simulink model "PathFollowing_4_29"  (R2023b)
settings: Solver=FixedStepAuto  StartTime=0  StopTime=inf  FixedStep=0.01  RelTol=1e-3
InitFcn:
  | InitParam_cs;
StopFcn:
  | plotTrack;
values from neighbouring files (symbols this model uses):
  B0 = [0,-30]    [InitParam_cs.m]
  lamda = 0.2573    [main.m]
  P0 = [0,0]    [InitParam_cs.m]    (also in SetWaypoints.m)
  u_c = 0.1    [main.m]
  U_d = i    [main.m]
  v_c = 0.1    [main.m]
  V_w = 1    [main.m]
  w_e1 = 0.8    [main.m]
  w_e2 = 0.8    [main.m]
  w_e6 = 0.8    [main.m]
  Waypoints = [100 0;200 0]    [InitParam_cs.m]    (also in SetWaypoints.m = [80 0;120 0])
  WPNum = size(Waypoints,1)    [InitParam_cs.m]    (also in SetWaypoints.m)
  Yaw0 = 0    [InitParam_cs.m]    (also in SetWaypoints.m)
libraries: simulink x9, cstblocks x3, slpidlib x2
settings Model: Creator=53549  LastModifiedBy=Xue
settings SolverCC: AlgebraicLoopSolver=TrustRegion
settings DataIOCC: SaveFormat=StructureWithTime  ReturnWorkspaceOutputs=off
settings OptimizationCC: BlockReduction=off  BufferReuse=off
settings DebuggingCC: AlgebraicLoopMsg=none  ArithmeticOperatorsInVariantConditions=warning
settings ModelReferenceCC: EnableRefExpFcnMdlSchedulingChecks=on
settings SFSimCC: SimUseLocalCustomCode=off  CustomCodeUndefinedFunction=UseInterfaceOnly
settings RTWCC: RTWUseLocalCustomCode=off  DLArmComputeVersion=19.05
settings CodeAppCC: StateflowObjectComments=on

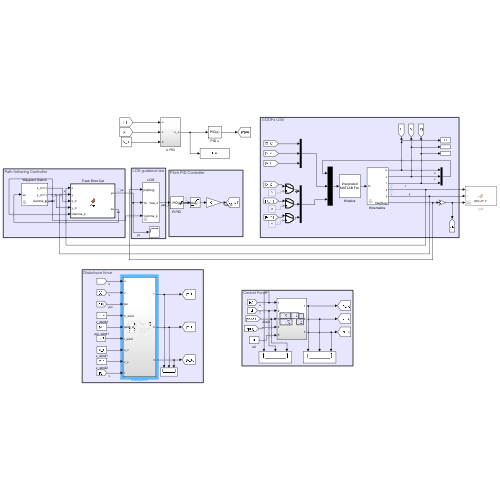
[thumbnail: Simulink's stored preview of the top-level diagram]
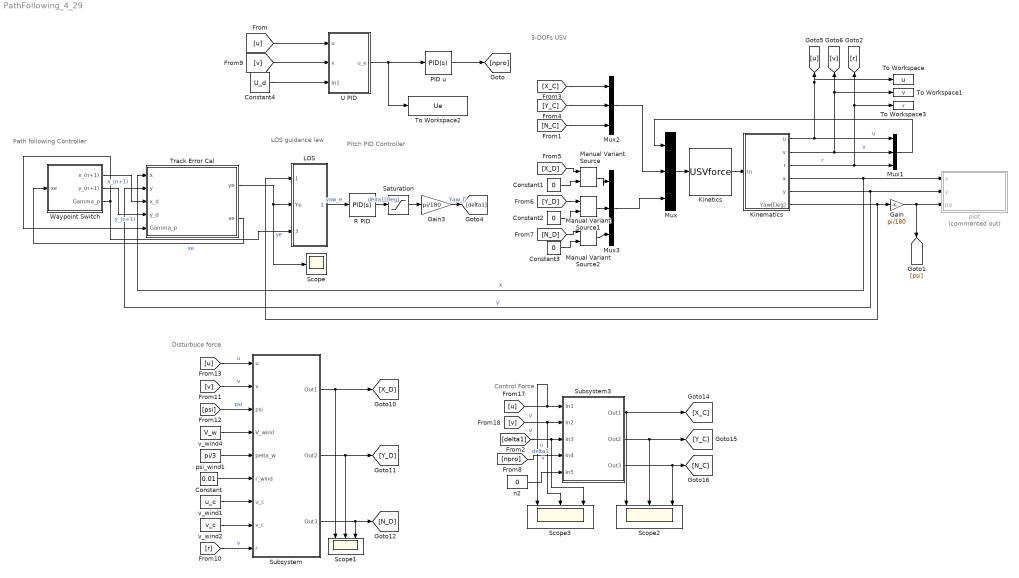
== system PathFollowing_4_29 ==
  note: LOS guidance law
  note: Disturbuce force
  note: v
  note: v
  note: Path following Controller
  note: 3-DOFs USV
  note: Control Force
  note: Pitch PID Controller
  Constant : Constant  Value=0.01
  Constant1 : Constant  Value=0
  Constant2 : Constant  Value=0
  Constant3 : Constant  Value=0
  Constant4 : Constant  Value=U_d
  Gain : Gain  Gain=pi/180
  Gain3 : Gain  Gain=pi/180
  "Kinematics " : Subsystem  mask{yawInit=Yaw0, u0=2, currentDir=45, currentVel=0.1}
      mask prompts: yawInit "Initial psi [Deg]"; u0 "Initial velocity [m/s]"; currentDir "current direction [Deg]"; currentVel "current velocity [m/s]"
      mask DialogControl DescGroupVar Prompt: Kinematics
      mask DialogControl DescTextVar Prompt: Set kinematics information: ASV initial state, flow disturance, etc
      mask DialogControl ParameterGroupVar Prompt: Initial state
      mask DialogControl Container3 Prompt: Flow
  Kinetics : MATLABFcn  MATLABFcn=USVforce  OutputDimensions=3  OutputSignalType=real
  LOS : Subsystem  mask{kp=260, ki=4, kd=25, losAlg=LOS, klos=4, KIlos=0}
      mask prompts: losAlg "Guidance Form"
      mask TypeOptions losAlg: LOS | ALOS
      mask DialogControl DescGroupVar Prompt: Path following control
      mask DialogControl DescTextVar Prompt: Please select the guidance law and set the parameters of heading autopilot and line of sight guidance.
      mask DialogControl ParameterGroupVar Prompt: Heading  Autopilot
      mask DialogControl Container3 Prompt: Guidance
  Manual Variant Source : simulink/Signal Routing/Manual Variant Source  NumChoices=2  LabelModeActiveChoice=V_1
  Manual Variant Source1 : simulink/Signal Routing/Manual Variant Source  NumChoices=2  LabelModeActiveChoice=V_1
  Manual Variant Source2 : simulink/Signal Routing/Manual Variant Source  NumChoices=2  LabelModeActiveChoice=V_1
  Mux{,1..3} (4 alike) : Mux  Inputs=3
  PID u : slpidlib/PID Controller  Controller=PID  Form=Parallel  TimeDomain=Continuous-time  UseExternalTs=off  SampleTime=-1  IntegratorMethod=Forward Euler  FilterMethod=Forward Euler  ControllerParametersSource=internal  P=1  I=1  UseKiTs=off  D=0  N=100  UseFilter=on  TunerSelectOption=Transfer Function Based (PID Tuner App)  InitialConditionSource=internal  InitialConditionForIntegrator=0  InitialConditionForFilter=0  DifferentiatorICPrevScaledInput=0  ExternalReset=none  TrackingMode=off  Kt=1  LimitOutput=off  SatLimitsSource=internal  UpperSaturationLimit=inf  LowerSaturationLimit=-inf  LinearizeAsGain=on  AntiWindupMode=none  Kb=1  LimitIntegrator=off  UpperIntegratorSaturationLimit=inf  LowerIntegratorSaturationLimit=-inf  POutMin=[]  POutMax=[]  IOutMin=[]  IOutMax=[]  DOutMin=[]  DOutMax=[]  NOutMin=[]  NOutMax=[]  SumOutMin=[]  SumOutMax=[]  SaturationOutMin=[]  SaturationOutMax=[]  PParamMin=[]  PParamMax=[]  IParamMin=[]  IParamMax=[]  DParamMin=[]  DParamMax=[]  NParamMin=[]  NParamMax=[]  KbParamMin=[]  KbParamMax=[]  KtParamMin=[]  KtParamMax=[]  KbOutMin=[]  KbOutMax=[]  KtOutMin=[]  KtOutMax=[]  IntegratorOutMin=[]  IntegratorOutMax=[]  FilterOutMin=[]  FilterOutMax=[]  SumI1OutMin=[]  SumI1OutMax=[]  SumI2OutMin=[]  SumI2OutMax=[]  SumI3OutMin=[]  SumI3OutMax=[]  SumI4OutMin=[]  SumI4OutMax=[]  SumDOutMin=[]  SumDOutMax=[]  DifferentiatorOutMin=[]  DifferentiatorOutMax=[]  FilterDiffOutCoefMin=[]  FilterDiffOutCoefMax=[]  ReciprocalOutMin=[]  ReciprocalOutMax=[]  SumDenOutMin=[]  SumDenOutMax=[]  SumNumOutMin=[]  SumNumOutMax=[]  DivideOutMin=[]  DivideOutMax=[]  UdiffTsProdOutMin=[]  UdiffTsProdOutMax=[]  NTsProdOutMin=[]  NTsProdOutMax=[]  UintegralTsProdOutMin=[]  UintegralTsProdOutMax=[]  UngainTsProdOutMin=[]  UngainTsProdOutMax=[]  ClampingZeroOutDataTypeStr=Inherit: Inherit via back propagation  ClampingZeroOutMin=[]  ClampingZeroOutMax=[]  FilterDenConstantOutDataTypeStr=Inherit: Inherit via back propagation  FilterDenConstantOutMin=[]  FilterDenConstantOutMax=[]  PCopyOutDataTypeStr=Inherit: Inherit via back propagation  PCopyOutMin=[]  PCopyOutMax=[]  NCopyOutDataTypeStr=Inherit: Inherit via back propagation  NCopyOutMin=[]  NCopyOutMax=[]  IntegratorContinuousStateAttributes=''  IntegratorStateMustResolveToSignalObject=off  IntegratorRTWStateStorageClass=Auto  FilterContinuousStateAttributes=''  FilterStateMustResolveToSignalObject=off  FilterRTWStateStorageClass=Auto  ParallelPVariant=InternalParameters  IdealPVariant=Disabled  IVariant=InternalParameters  DVariant=InternalParameters  IntegratorVariant=Continuous  SatVariant=Disabled  AWVariant=Passthrough  PCopyVariant=Disabled  TRVariant=Disabled  FdbkBlocksVariant=Forward  IdealPFdbkVariant=Disabled  SatFdbkVariant=Disabled  DerivativeFilterVariant=ContFilter  NVariant=InternalParameters  NCopyVariant=Disabled  FilterICVariant=InternalICsFilter  IntegratorICVariant=InternalICs  ExternalResetVariant=Disabled  TRSumVariant=Passthrough  SumFdbkVariant=Disabled  SumVariant=Sum_PID  TsampFilterVariant=InternalTs  TsampNgainVariant=Passthrough  TsampIntegralVariant=Disabled_SignalSpec  ExternalSaturationOutDataTypeStr=Inherit: Same as second input
  "R PID " : slpidlib/PID Controller  Controller=PID  Form=Parallel  TimeDomain=Continuous-time  UseExternalTs=off  SampleTime=-1  IntegratorMethod=Forward Euler  FilterMethod=Forward Euler  ControllerParametersSource=internal  P=250  I=4  UseKiTs=off  D=25  N=10  UseFilter=on  TunerSelectOption=Transfer Function Based (PID Tuner App)  InitialConditionSource=internal  InitialConditionForIntegrator=0  InitialConditionForFilter=0  DifferentiatorICPrevScaledInput=0  ExternalReset=none  TrackingMode=off  Kt=1  LimitOutput=on  SatLimitsSource=internal  UpperSaturationLimit=20  LowerSaturationLimit=-20  LinearizeAsGain=on  AntiWindupMode=none  Kb=1  LimitIntegrator=off  UpperIntegratorSaturationLimit=inf  LowerIntegratorSaturationLimit=-inf  POutMin=[]  POutMax=[]  IOutMin=[]  IOutMax=[]  DOutMin=[]  DOutMax=[]  NOutMin=[]  NOutMax=[]  SumOutMin=[]  SumOutMax=[]  SaturationOutMin=[]  SaturationOutMax=[]  PParamMin=[]  PParamMax=[]  IParamMin=[]  IParamMax=[]  DParamMin=[]  DParamMax=[]  NParamMin=[]  NParamMax=[]  KbParamMin=[]  KbParamMax=[]  KtParamMin=[]  KtParamMax=[]  KbOutMin=[]  KbOutMax=[]  KtOutMin=[]  KtOutMax=[]  IntegratorOutMin=[]  IntegratorOutMax=[]  FilterOutMin=[]  FilterOutMax=[]  SumI1OutMin=[]  SumI1OutMax=[]  SumI2OutMin=[]  SumI2OutMax=[]  SumI3OutMin=[]  SumI3OutMax=[]  SumI4OutMin=[]  SumI4OutMax=[]  SumDOutMin=[]  SumDOutMax=[]  DifferentiatorOutMin=[]  DifferentiatorOutMax=[]  FilterDiffOutCoefMin=[]  FilterDiffOutCoefMax=[]  ReciprocalOutMin=[]  ReciprocalOutMax=[]  SumDenOutMin=[]  SumDenOutMax=[]  SumNumOutMin=[]  SumNumOutMax=[]  DivideOutMin=[]  DivideOutMax=[]  UdiffTsProdOutMin=[]  UdiffTsProdOutMax=[]  NTsProdOutMin=[]  NTsProdOutMax=[]  UintegralTsProdOutMin=[]  UintegralTsProdOutMax=[]  UngainTsProdOutMin=[]  UngainTsProdOutMax=[]  ClampingZeroOutDataTypeStr=Inherit: Inherit via back propagation  ClampingZeroOutMin=[]  ClampingZeroOutMax=[]  FilterDenConstantOutDataTypeStr=Inherit: Inherit via back propagation  FilterDenConstantOutMin=[]  FilterDenConstantOutMax=[]  PCopyOutDataTypeStr=Inherit: Inherit via back propagation  PCopyOutMin=[]  PCopyOutMax=[]  NCopyOutDataTypeStr=Inherit: Inherit via back propagation  NCopyOutMin=[]  NCopyOutMax=[]  IntegratorContinuousStateAttributes=''  IntegratorStateMustResolveToSignalObject=off  IntegratorRTWStateStorageClass=Auto  FilterContinuousStateAttributes=''  FilterStateMustResolveToSignalObject=off  FilterRTWStateStorageClass=Auto  ParallelPVariant=InternalParameters  IdealPVariant=Disabled  IVariant=InternalParameters  DVariant=InternalParameters  IntegratorVariant=Continuous  SatVariant=Enabled  AWVariant=Passthrough  PCopyVariant=Disabled  TRVariant=Disabled  FdbkBlocksVariant=Forward  IdealPFdbkVariant=Disabled  SatFdbkVariant=Disabled  DerivativeFilterVariant=ContFilter  NVariant=InternalParameters  NCopyVariant=Disabled  FilterICVariant=InternalICsFilter  IntegratorICVariant=InternalICs  ExternalResetVariant=Disabled  TRSumVariant=Passthrough  SumFdbkVariant=Disabled  SumVariant=Sum_PID  TsampFilterVariant=InternalTs  TsampNgainVariant=Passthrough  TsampIntegralVariant=Disabled_SignalSpec  ExternalSaturationOutDataTypeStr=Inherit: Same as second input
  Saturation : Saturate  UpperLimit=60  LowerLimit=-60
  Scope : Scope
  Scope1 : Scope  NumInputPorts=3
  Scope2 : Scope  NumInputPorts=3
  Scope3 : Scope  NumInputPorts=3
  Subsystem : Subsystem
  Subsystem3 : Subsystem
  To Workspace : ToWorkspace  VariableName=u  SampleTime=-1
  To Workspace1 : ToWorkspace  VariableName=v  SampleTime=-1
  To Workspace2 : ToWorkspace  VariableName=Ue  SaveFormat=Timeseries  SampleTime=-1
  To Workspace3 : ToWorkspace  VariableName=r  SampleTime=-1
  Track Error Cal : MATLAB Function  TreatAsAtomicUnit=on
  U PID : Subsystem
  Waypoint Switch : Subsystem  mask{WP=Waypoints, WPNum=WPNum, xm=10}
      mask prompts: WP "Waypoints"; WPNum "Waypoints Sum"
      mask DialogControl DescGroupVar Prompt: Task Waypoints
      mask DialogControl DescTextVar Prompt: Please set waypoints and the sum.
  n2 : Constant  Value=0
  plot : MATLAB Function  Commented=on  TreatAsAtomicUnit=on
  psi_wind1 : Constant  Value=pi/3
  v_wind1 : Constant  Value=u_c
  v_wind2 : Constant  Value=v_c
  v_wind4 : Constant  Value=V_w
  wires:
  Kinetics/1 -> "Kinematics "/1(In)
  Mux/1 -> Kinetics/1
  "Kinematics "/6(Yaw[Deg]) -> LOS/1(psi[Deg]), Gain/1
  "Kinematics "/1(u) -> Mux1/1, To Workspace/1, [u]  "u"
  "Kinematics "/2(v) -> Mux1/2, To Workspace1/1, [v]  "v"
  "Kinematics "/3(r) -> To Workspace3/1, [r], Mux1/3  "r"
  Mux1/1 -> Mux/1
  "Kinematics "/4(x) -> plot/1(x), Track Error Cal/1(x)  "x"
  "Kinematics "/5(y) -> plot/2(y), Track Error Cal/2(y)  "y"
  [Y_C] -> Mux2/2
  Track Error Cal/1(ye) -> Scope/1, LOS/2(Ye)  "ye"
  Track Error Cal/2(xe) -> Waypoint Switch/1(xe)  "xe"
  Waypoint Switch/1(x_(n+1)) -> Track Error Cal/3(x_d)  "x_(n+1)"
  Waypoint Switch/2(y_(n+1)) -> Track Error Cal/4(y_d)  "y_(n+1)"
  Waypoint Switch/3(Gamma_p) -> Track Error Cal/5(Gamma_p), LOS/3(Gamma_p)
  Gain/1 -> plot/3(psi), [psi]
  [X_C] -> Mux2/1
  U PID/1(u_e) -> To Workspace2/1, PID u/1
  LOS/1(Yaw_e) -> "R PID "/1  "yaw_e"
  [N_C] -> Mux2/3
  Subsystem3/2(Out2) -> Scope2/2, [Y_C]
  Subsystem3/3(Out3) -> Scope2/3, [N_C]
  Subsystem3/1(Out1) -> Scope2/1, [X_C]
  [u] -> Scope3/1, Subsystem3/1(In1)  "u"
  [v] -> Scope3/2, Subsystem3/2(In2)  "v"
  [delta1] -> Scope3/3, Subsystem3/3(In3)  "delta1"
  [npro] -> Subsystem3/4(In4)
  n2/1 -> Subsystem3/5(In5)
  Mux2/1 -> Mux/2
  Mux3/1 -> Mux/3
  [X_D] -> Manual Variant Source/1
  [u] -> Subsystem/1(u)  "u"
  [v] -> Subsystem/2(v)  "v"
  [psi] -> Subsystem/3(psi)  "psi"
  v_wind4/1 -> Subsystem/4(V_wind)
  psi_wind1/1 -> Subsystem/5(peita_w)
  Constant/1 -> Subsystem/6(r_wind)
  Subsystem/1(Out1) -> [X_D], Scope1/1
  Subsystem/2(Out2) -> [Y_D], Scope1/2
  Subsystem/3(Out3) -> Scope1/3, [N_D]
  Manual Variant Source/1 -> Mux3/1
  Constant1/1 -> Manual Variant Source/2
  Constant2/1 -> Manual Variant Source1/2
  [Y_D] -> Manual Variant Source1/1
  Manual Variant Source1/1 -> Mux3/2
  Constant3/1 -> Manual Variant Source2/2
  Manual Variant Source2/1 -> Mux3/3
  [N_D] -> Manual Variant Source2/1
  PID u/1 -> [npro]
  Saturation/1 -> Gain3/1
  "R PID "/1 -> Saturation/1  "delta1[Deg]"
  Gain3/1 -> [delta1]  "Yaw_D"
  [u] -> U PID/1(u)
  [v] -> U PID/2(v)
  Constant4/1 -> U PID/3(In1)
  v_wind1/1 -> Subsystem/7(u_c)
  v_wind2/1 -> Subsystem/8(v_c)
  [r] -> Subsystem/9(r)  "v"

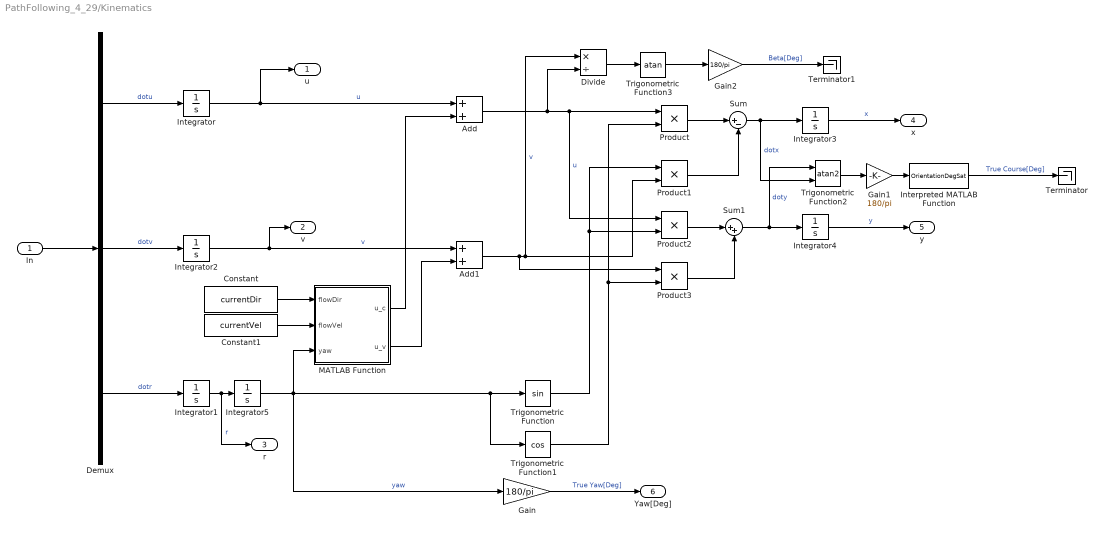
== system PathFollowing_4_29/Kinematics  ==
  In : Inport
  Add : Sum
  Add1 : Sum
  Constant : Constant  Value=currentDir
  Constant1 : Constant  Value=currentVel
  Demux : Demux  Outputs=3
  Divide : Product  Inputs=*/
  Gain : Gain  Gain=180/pi
  Gain1 : Gain  Gain=180/pi
  Gain2 : Gain  Gain=180/pi
  Integrator : Integrator  InitialCondition=u0
  Integrator1 : Integrator
  Integrator2 : Integrator
  Integrator3 : Integrator  InitialCondition=B0(1)
  Integrator4 : Integrator  InitialCondition=B0(2)
  Integrator5 : Integrator  InitialCondition=yawInit*pi/180  WrapState=on  WrappedStateUpperValue=6.2832  WrappedStateLowerValue=0
  Interpreted MATLAB Function : MATLABFcn  MATLABFcn=OrientationDegSat
  MATLAB Function : MATLAB Function  TreatAsAtomicUnit=on
  Product{,1..3} (4 alike) : Product
  Sum : Sum  Inputs=|+-
  Sum1 : Sum  Inputs=|++
  Terminator : Terminator
  Terminator1 : Terminator
  Trigonometric Function : Trigonometry
  Trigonometric Function1 : Trigonometry  Operator=cos
  Trigonometric Function2 : Trigonometry  Operator=atan2
  Trigonometric Function3 : Trigonometry  Operator=atan
  u : Outport
  v : Outport  Port=2
  r : Outport  Port=3
  x : Outport  Port=4
  y : Outport  Port=5
  Yaw[Deg] : Outport  Port=6
  wires:
  Integrator2/1 -> Add1/1, v/1  "v"
  Integrator3/1 -> x/1  "x"
  Product2/1 -> Sum1/1
  Product1/1 -> Sum/2
  Demux/1 -> Integrator/1  "dotu"
  Demux/2 -> Integrator2/1  "dotv"
  Demux/3 -> Integrator1/1  "dotr"
  Trigonometric Function1/1 -> Product/2, Product3/2
  Product/1 -> Sum/1
  Product3/1 -> Sum1/2
  In/1 -> Demux/1
  Integrator4/1 -> y/1  "y"
  Sum/1 -> Trigonometric Function2/2, Integrator3/1  "dotx"
  Integrator/1 -> Add/1, u/1  "u"
  Trigonometric Function/1 -> Product1/1, Product2/2
  Sum1/1 -> Trigonometric Function2/1, Integrator4/1  "doty"
  Integrator1/1 -> r/1, Integrator5/1  "r"
  Integrator5/1 -> Gain/1, MATLAB Function/3(yaw), Trigonometric Function1/1, Trigonometric Function/1  "yaw"
  Gain/1 -> Yaw[Deg]/1  "True Yaw[Deg]"
  Constant/1 -> MATLAB Function/1(flowDir)
  Constant1/1 -> MATLAB Function/2(flowVel)
  Add/1 -> Product/1, Product2/1, Divide/2  "u"
  MATLAB Function/1(u_c) -> Add/2
  MATLAB Function/2(u_v) -> Add1/2
  Add1/1 -> Divide/1, Product1/2, Product3/1  "v"
  Trigonometric Function2/1 -> Gain1/1
  Gain1/1 -> Interpreted MATLAB Function/1
  Interpreted MATLAB Function/1 -> Terminator/1  "True Course[Deg]"
  Gain2/1 -> Terminator1/1  "Beta[Deg]"
  Divide/1 -> Trigonometric Function3/1
  Trigonometric Function3/1 -> Gain2/1

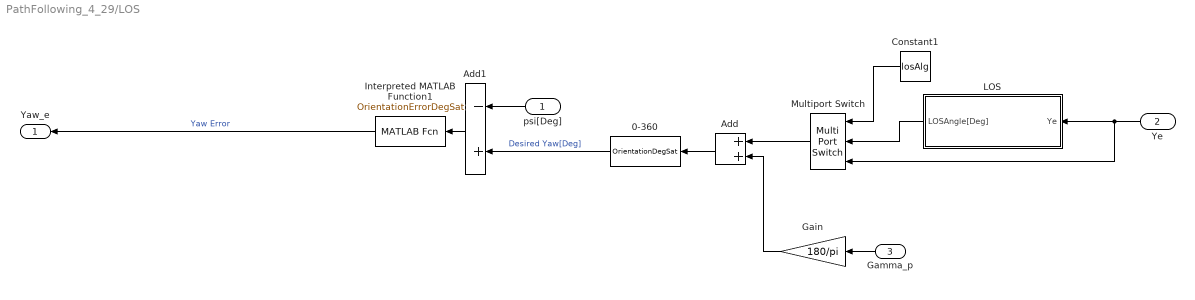
== system PathFollowing_4_29/LOS ==
  psi[Deg] : Inport
  Ye : Inport  Port=2
  Gamma_p : Inport  Port=3
  0-360 : MATLABFcn  MATLABFcn=OrientationDegSat  OutputDimensions=1
  Add : Sum
  Add1 : Sum  Inputs=-+
  Constant1 : Constant  Value=losAlg
  Gain : Gain  Gain=180/pi
  Interpreted MATLAB Function1 : MATLABFcn  MATLABFcn=OrientationErrorDegSat  OutputDimensions=1
  LOS : Subsystem
  Multiport Switch : MultiPortSwitch  Inputs=2  SaturateOnIntegerOverflow=off  InputSameDT=off
  Yaw_e : Outport
  wires:
  psi[Deg]/1 -> Add1/1
  Add1/1 -> Interpreted MATLAB Function1/1
  0-360/1 -> Add1/2  "Desired Yaw[Deg]"
  Ye/1 -> Multiport Switch/3, LOS/1(Ye)
  LOS/1(LOSAngle[Deg]) -> Multiport Switch/2
  Multiport Switch/1 -> Add/1
  Constant1/1 -> Multiport Switch/1
  Gamma_p/1 -> Gain/1
  Add/1 -> 0-360/1
  Gain/1 -> Add/2
  Interpreted MATLAB Function1/1 -> Yaw_e/1  "Yaw Error"

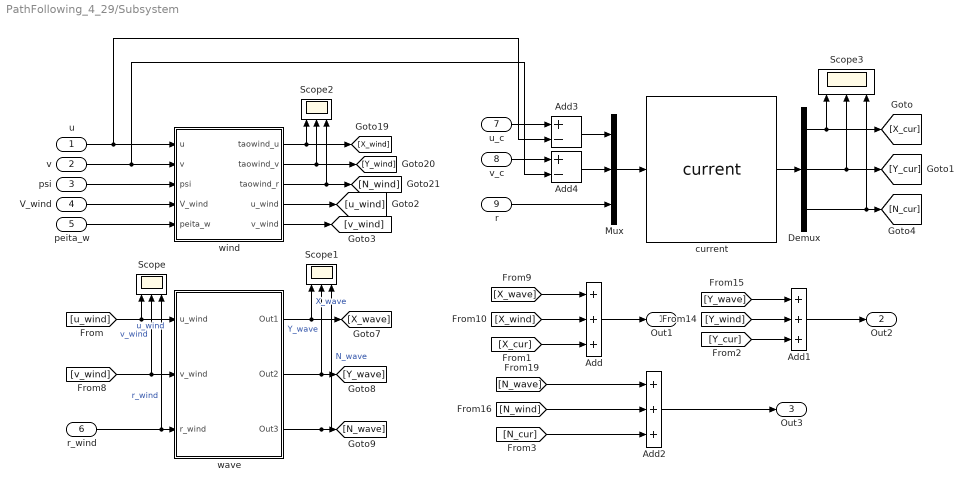
== system PathFollowing_4_29/Subsystem ==
  u : Inport
  v : Inport  Port=2
  psi : Inport  Port=3
  V_wind : Inport  Port=4
  peita_w : Inport  Port=5
  r_wind : Inport  Port=6
  u_c : Inport  Port=7
  v_c : Inport  Port=8
  r : Inport  Port=9
  Add : Sum  Inputs=+++
  Add1 : Sum  Inputs=+++
  Add2 : Sum  Inputs=+++
  Add3 : Sum  Inputs=+-
  Add4 : Sum  Inputs=+-
  Demux : Demux  Outputs=3
  Mux : Mux  Inputs=3
  Scope{,1..3} (4 alike) : Scope  NumInputPorts=3
  current : MATLABFcn  MATLABFcn=current
  wave : Subsystem
  wind : Subsystem
  Out1 : Outport
  Out2 : Outport  Port=2
  Out3 : Outport  Port=3
  wires:
  [X_wind] -> Add/2
  wind/4(u_wind) -> [u_wind]
  wind/3(taowind_r) -> Scope2/3, [N_wind]
  [Y_wave] -> Add1/1
  wind/2(taowind_v) -> Scope2/2, [Y_wind]
  wave/1(Out1) -> Scope1/1, [X_wave]  "X_wave"
  wind/1(taowind_u) -> Scope2/1, [X_wind]
  [u_wind] -> wave/1(u_wind), Scope/1  "u_wind"
  wind/5(v_wind) -> [v_wind]
  [Y_wind] -> Add1/2
  [X_wave] -> Add/1
  v/1 -> Add4/2, wind/2(v)
  [N_wave] -> Add2/1
  [N_wind] -> Add2/2
  [v_wind] -> wave/2(v_wind), Scope/2  "v_wind"
  wave/3(Out3) -> Scope1/3, [N_wave]  "N_wave"
  wave/2(Out2) -> Scope1/2, [Y_wave]  "Y_wave"
  V_wind/1 -> wind/4(V_wind)
  Add2/1 -> Out3/1
  u/1 -> Add3/2, wind/1(u)
  peita_w/1 -> wind/5(peita_w)
  psi/1 -> wind/3(psi)
  Add/1 -> Out1/1
  Add1/1 -> Out2/1
  r_wind/1 -> wave/3(r_wind), Scope/3  "r_wind"
  Mux/1 -> current/1
  current/1 -> Demux/1
  Demux/2 -> Scope3/2, [Y_cur]
  Demux/3 -> Scope3/3, [N_cur]
  u_c/1 -> Add3/1
  v_c/1 -> Add4/1
  Add3/1 -> Mux/1
  Add4/1 -> Mux/2
  r/1 -> Mux/3
  Demux/1 -> [X_cur], Scope3/1
  [X_cur] -> Add/3
  [Y_cur] -> Add1/3
  [N_cur] -> Add2/3

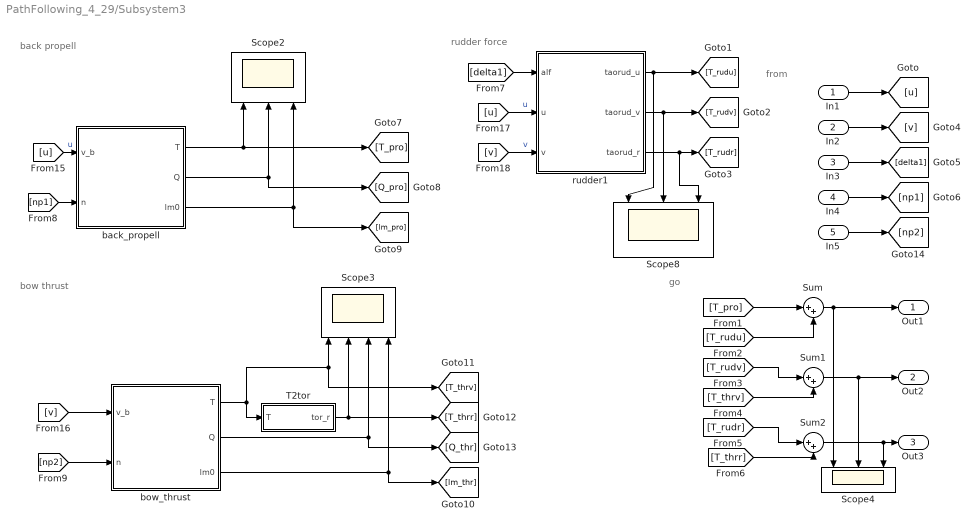
== system PathFollowing_4_29/Subsystem3 ==
  note: from
  note: go
  note: back propell
  note: bow thrust
  note: rudder force
  In1 : Inport
  In2 : Inport  Port=2
  In3 : Inport  Port=3
  In4 : Inport  Port=4
  In5 : Inport  Port=5
  Scope2 : Scope  NumInputPorts=3
  Scope3 : Scope  NumInputPorts=4
  Scope4 : Scope  NumInputPorts=3
  Scope8 : Scope  NumInputPorts=3
  Sum : Sum  Inputs=|++
  Sum1 : Sum  Inputs=|++
  Sum2 : Sum  Inputs=|++
  T2tor : MATLAB Function  TreatAsAtomicUnit=on
  back_propell : MATLAB Function  TreatAsAtomicUnit=on
  bow_thrust : MATLAB Function  TreatAsAtomicUnit=on
  rudder1 : MATLAB Function  TreatAsAtomicUnit=on
  Out1 : Outport
  Out2 : Outport  Port=2
  Out3 : Outport  Port=3
  wires:
  [T_thrv] -> Sum1/2
  [T_rudv] -> Sum1/1
  [T_rudr] -> Sum2/1
  Sum2/1 -> Out3/1, Scope4/3
  Sum/1 -> Out1/1, Scope4/1
  Sum1/1 -> Out2/1, Scope4/2
  [T_rudu] -> Sum/2
  [T_thrr] -> Sum2/2
  [T_pro] -> Sum/1
  back_propell/2(Q) -> [Q_pro], Scope2/2
  back_propell/1(T) -> Scope2/1, [T_pro]
  [u] -> back_propell/1(v_b)  "u"
  back_propell/3(lm0) -> [lm_pro], Scope2/3
  [np1] -> back_propell/2(n)
  T2tor/1(tor_r) -> [T_thrr], Scope3/2
  bow_thrust/2(Q) -> [Q_thr], Scope3/3
  bow_thrust/3(lm0) -> [lm_thr], Scope3/4
  bow_thrust/1(T) -> [T_thrv], Scope3/1, T2tor/1(T)
  [np2] -> bow_thrust/2(n)
  [v] -> bow_thrust/1(v_b)
  [delta1] -> rudder1/1(alf)
  [v] -> rudder1/3(v)  "v"
  [u] -> rudder1/2(u)  "u"
  rudder1/1(taorud_u) -> [T_rudu], Scope8/1
  rudder1/3(taorud_r) -> Scope8/3, [T_rudr]
  rudder1/2(taorud_v) -> [T_rudv], Scope8/2
  In1/1 -> [u]
  In2/1 -> [v]
  In3/1 -> [delta1]
  In4/1 -> [np1]
  In5/1 -> [np2]

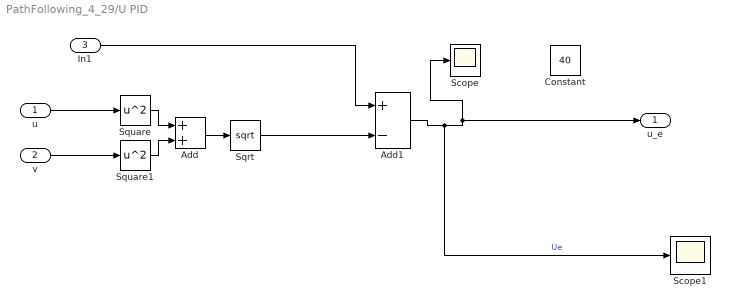
== system PathFollowing_4_29/U PID ==
  u : Inport
  v : Inport  Port=2
  In1 : Inport  Port=3
  Add : Sum
  Add1 : Sum  Inputs=+-
  Constant : Constant  Value=40
  Scope : Scope
  Scope1 : Scope
  Sqrt : Sqrt
  Square : Math  Operator=square  SignedPower=on  RndMeth=Zero
  Square1 : Math  Operator=square  SignedPower=on  RndMeth=Zero
  u_e : Outport
  wires:
  Square/1 -> Add/1
  Add/1 -> Sqrt/1
  u/1 -> Square/1
  Square1/1 -> Add/2
  In1/1 -> Add1/1
  Sqrt/1 -> Add1/2
  v/1 -> Square1/1
  Add1/1 -> Scope1/1, u_e/1, Scope/1  "Ue"

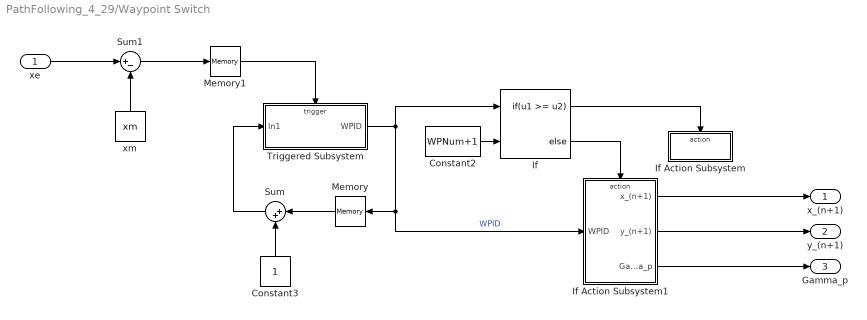
== system PathFollowing_4_29/Waypoint Switch ==
  xe : Inport
  Constant2 : Constant  Value=WPNum+1
  Constant3 : Constant
  If : If  NumInputs=2  IfExpression=u1 >= u2
  If Action Subsystem : Subsystem  TreatAsAtomicUnit=on
  If Action Subsystem1 : Subsystem  TreatAsAtomicUnit=on
  Memory : Memory  InitialCondition=1  InheritSampleTime=on
  Memory1 : Memory  InitialCondition=5  InheritSampleTime=on
  Sum : Sum  Inputs=|++
  Sum1 : Sum  Inputs=|+-
  Triggered Subsystem : Subsystem  TreatAsAtomicUnit=on
  xm : Constant  Value=xm
  x_(n+1) : Outport
  y_(n+1) : Outport  Port=2
  Gamma_p : Outport  Port=3
  wires:
  If Action Subsystem1/2(y_(n+1)) -> y_(n+1)/1
  Constant2/1 -> If/2
  If Action Subsystem1/3(Gamma_p) -> Gamma_p/1
  Sum1/1 -> Memory1/1
  Memory/1 -> Sum/1
  If/2 -> If Action Subsystem1/Action
  xe/1 -> Sum1/1
  Sum/1 -> Triggered Subsystem/1(In1)
  Constant3/1 -> Sum/2
  If Action Subsystem1/1(x_(n+1)) -> x_(n+1)/1
  Triggered Subsystem/1(WPID) -> If/1, If Action Subsystem1/1(WPID), Memory/1  "WPID"
  xm/1 -> Sum1/2
  If/1 -> If Action Subsystem/Action
  Memory1/1 -> Triggered Subsystem/Trigger

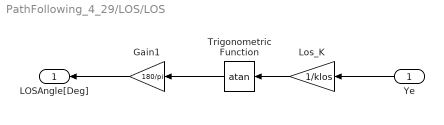
== system PathFollowing_4_29/LOS/LOS ==
  Ye : Inport
  Gain1 : Gain  Gain=180/pi
  Los_K : Gain  Gain=1/klos
  Trigonometric Function : Trigonometry  Operator=atan
  LOSAngle[Deg] : Outport
  wires:
  Los_K/1 -> Trigonometric Function/1
  Ye/1 -> Los_K/1
  Gain1/1 -> LOSAngle[Deg]/1
  Trigonometric Function/1 -> Gain1/1

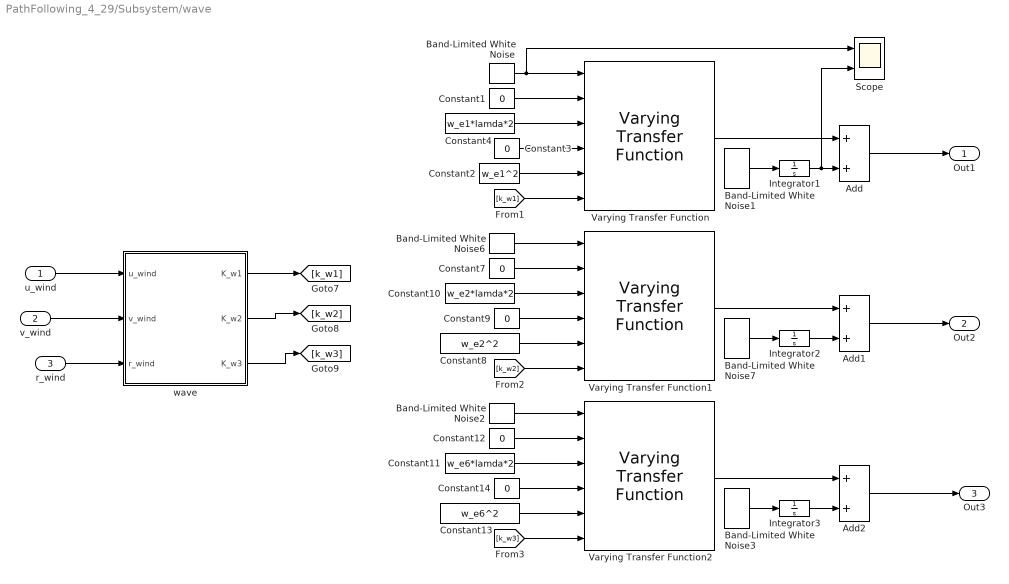
== system PathFollowing_4_29/Subsystem/wave ==
  u_wind : Inport
  v_wind : Inport  Port=2
  r_wind : Inport  Port=3
  Add : Sum
  Add1 : Sum
  Add2 : Sum
  Band-Limited White Noise : simulink/Sources/Band-Limited White Noise  Cov=[0.1]  Ts=0.1  seed=[23345]
  Band-Limited White Noise1 : simulink/Sources/Band-Limited White Noise  Cov=[0.1]  Ts=0.1  seed=[23327]
  Band-Limited White Noise2 : simulink/Sources/Band-Limited White Noise  Cov=[0.1]  Ts=0.1  seed=[23310]
  Band-Limited White Noise3 : simulink/Sources/Band-Limited White Noise  Cov=[0.1]  Ts=0.1  seed=[23301]
  Band-Limited White Noise6 : simulink/Sources/Band-Limited White Noise  Cov=[0.1]  Ts=0.1  seed=[23367]
  Band-Limited White Noise7 : simulink/Sources/Band-Limited White Noise  Cov=[0.1]  Ts=0.1  seed=[23328]
  Constant{1,3,7,9,12,14} (6 alike) : Constant  Value=0
  Constant10 : Constant  Value=w_e2*lamda*2
  Constant11 : Constant  Value=w_e6*lamda*2
  Constant13 : Constant  Value=w_e6^2
  Constant2 : Constant  Value=w_e1^2
  Constant4 : Constant  Value=w_e1*lamda*2
  Constant8 : Constant  Value=w_e2^2
  Integrator1 : Integrator
  Integrator2 : Integrator
  Integrator3 : Integrator
  Scope : Scope  NumInputPorts=2
  Varying Transfer Function : cstblocks/Linear Parameter Varying/Varying Transfer Function  N=2  Feedthrough=on
  Varying Transfer Function1 : cstblocks/Linear Parameter Varying/Varying Transfer Function  N=2  Feedthrough=on
  Varying Transfer Function2 : cstblocks/Linear Parameter Varying/Varying Transfer Function  N=2  Feedthrough=on
  wave : MATLAB Function  TreatAsAtomicUnit=on
  Out1 : Outport
  Out2 : Outport  Port=2
  Out3 : Outport  Port=3
  wires:
  wave/2(K_w2) -> [k_w2]
  Band-Limited White Noise1/1 -> Integrator1/1
  wave/3(K_w3) -> [k_w3]
  r_wind/1 -> wave/3(r_wind)
  Constant9/1 -> Varying Transfer Function1/4
  Band-Limited White Noise7/1 -> Integrator2/1
  Constant3/1 -> Varying Transfer Function/4
  Band-Limited White Noise3/1 -> Integrator3/1
  [k_w1] -> Varying Transfer Function/6
  Constant14/1 -> Varying Transfer Function2/4
  Constant4/1 -> Varying Transfer Function/3
  Constant12/1 -> Varying Transfer Function2/2
  wave/1(K_w1) -> [k_w1]
  Band-Limited White Noise/1 -> Scope/1, Varying Transfer Function/1
  v_wind/1 -> wave/2(v_wind)
  Integrator2/1 -> Add1/2
  Constant1/1 -> Varying Transfer Function/2
  Constant2/1 -> Varying Transfer Function/5
  [k_w2] -> Varying Transfer Function1/6
  Integrator1/1 -> Scope/2, Add/2
  Band-Limited White Noise6/1 -> Varying Transfer Function1/1
  Varying Transfer Function/1 -> Add/1
  Constant8/1 -> Varying Transfer Function1/5
  Varying Transfer Function1/1 -> Add1/1
  Constant11/1 -> Varying Transfer Function2/3
  Constant7/1 -> Varying Transfer Function1/2
  Constant10/1 -> Varying Transfer Function1/3
  [k_w3] -> Varying Transfer Function2/6
  Constant13/1 -> Varying Transfer Function2/5
  Varying Transfer Function2/1 -> Add2/1
  Band-Limited White Noise2/1 -> Varying Transfer Function2/1
  Integrator3/1 -> Add2/2
  Add/1 -> Out1/1
  Add1/1 -> Out2/1
  Add2/1 -> Out3/1
  u_wind/1 -> wave/1(u_wind)

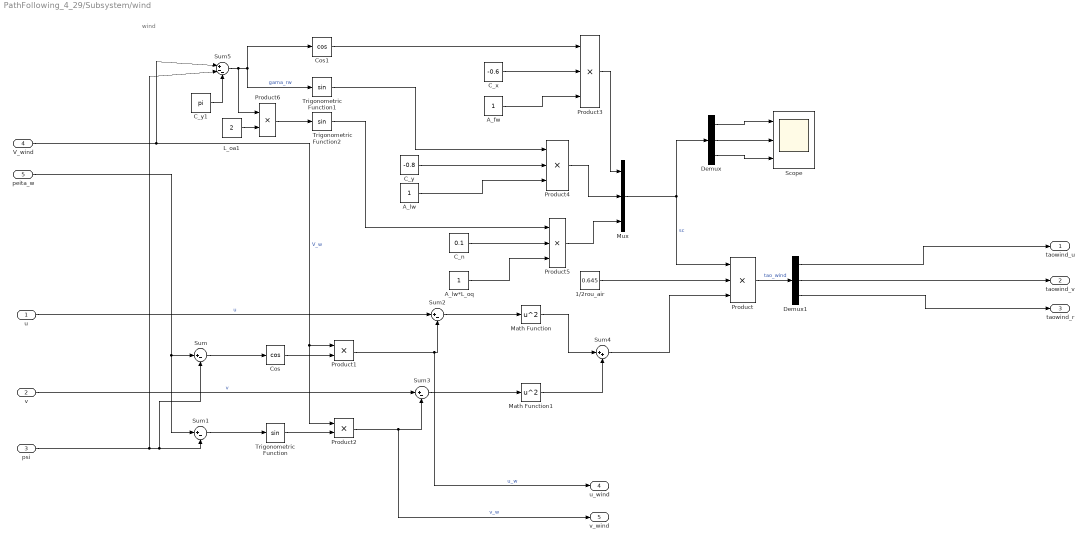
== system PathFollowing_4_29/Subsystem/wind ==
  note: wind
  u : Inport
  v : Inport  Port=2
  psi : Inport  Port=3
  V_wind : Inport  Port=4
  peita_w : Inport  Port=5
  1/2rou_air : Constant  Value=0.645
  A_fw : Constant
  A_lw : Constant
  A_lw*L_oq : Constant
  C_n : Constant  Value=0.1
  C_x : Constant  Value=-0.6
  C_y : Constant  Value=-0.8
  C_y1 : Constant  Value=pi
  Cos : Trigonometry  Operator=cos
  Cos1 : Trigonometry  Operator=cos
  Demux : Demux  Outputs=3
  Demux1 : Demux  Outputs=3
  L_oa1 : Constant  Value=2
  Math Function : Math  Operator=square  SignedPower=on
  Math Function1 : Math  Operator=square  SignedPower=on
  Mux : Mux  Inputs=3
  Product{,3..5} (4 alike) : Product  Inputs=3
  Product1 : Product
  Product2 : Product
  Product6 : Product
  Scope : Scope  NumInputPorts=3
  Sum{,1..3} (4 alike) : Sum  Inputs=|+-
  Sum4 : Sum  Inputs=|++
  Sum5 : Sum  Inputs=|+--
  Trigonometric Function : Trigonometry
  Trigonometric Function1 : Trigonometry
  Trigonometric Function2 : Trigonometry
  taowind_u : Outport  VectorParamsAs1DForOutWhenUnconnected=off
  taowind_v : Outport  Port=2  VectorParamsAs1DForOutWhenUnconnected=off
  taowind_r : Outport  Port=3  VectorParamsAs1DForOutWhenUnconnected=off
  u_wind : Outport  Port=4  VectorParamsAs1DForOutWhenUnconnected=off
  v_wind : Outport  Port=5  VectorParamsAs1DForOutWhenUnconnected=off
  wires:
  Demux1/3 -> taowind_r/1
  Demux1/1 -> taowind_u/1
  Demux1/2 -> taowind_v/1
  Product/1 -> Demux1/1  "tao_wind"
  Demux/3 -> Scope/3
  Demux/1 -> Scope/1
  Sum1/1 -> Trigonometric Function/1
  Product5/1 -> Mux/3
  1/2rou_air/1 -> Product/2
  Math Function1/1 -> Sum4/2
  Math Function/1 -> Sum4/1
  Sum3/1 -> Math Function1/1
  Trigonometric Function/1 -> Product2/2
  Product3/1 -> Mux/1
  Cos/1 -> Product1/2
  Product2/1 -> v_wind/1, Sum3/2  "v_w"
  Sum4/1 -> Product/3
  V_wind/1 -> Sum5/1, Product2/1, Product1/1  "V_w"
  u/1 -> Sum2/1  "u"
  Mux/1 -> Product/1, Demux/1  "sc"
  Product1/1 -> u_wind/1, Sum2/2  "u_w"
  psi/1 -> Sum5/2, Sum/2, Sum1/2
  Sum2/1 -> Math Function/1
  Product4/1 -> Mux/2
  v/1 -> Sum3/1  "v"
  Sum/1 -> Cos/1
  Demux/2 -> Scope/2
  peita_w/1 -> Sum1/1, Sum/1
  C_y1/1 -> Sum5/3
  Sum5/1 -> Product6/1, Trigonometric Function1/1, Cos1/1  "gama_rw"
  L_oa1/1 -> Product6/2
  Product6/1 -> Trigonometric Function2/1
  Cos1/1 -> Product3/1
  C_x/1 -> Product3/2
  A_fw/1 -> Product3/3
  C_y/1 -> Product4/2
  A_lw/1 -> Product4/3
  Trigonometric Function1/1 -> Product4/1
  C_n/1 -> Product5/2
  A_lw*L_oq/1 -> Product5/3
  Trigonometric Function2/1 -> Product5/1

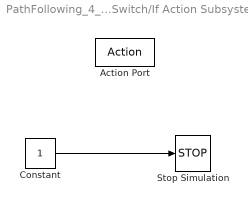
== system PathFollowing_4_29/Waypoint Switch/If Action Subsystem ==
  Action Port : ActionPort  ActionPortLabel=if(u1 >= u2)
  Constant : Constant
  Stop Simulation : Stop
  wires:
  Constant/1 -> Stop Simulation/1

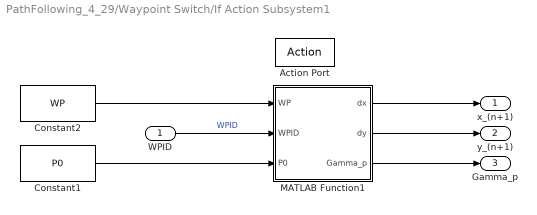
== system PathFollowing_4_29/Waypoint Switch/If Action Subsystem1 ==
  WPID : Inport
  Action Port : ActionPort  ActionPortLabel=else
  Constant1 : Constant  Value=P0
  Constant2 : Constant  Value=WP
  MATLAB Function1 : MATLAB Function  TreatAsAtomicUnit=on
  x_(n+1) : Outport
  y_(n+1) : Outport  Port=2
  Gamma_p : Outport  Port=3
  wires:
  MATLAB Function1/3(Gamma_p) -> Gamma_p/1
  MATLAB Function1/1(dx) -> x_(n+1)/1
  MATLAB Function1/2(dy) -> y_(n+1)/1
  Constant2/1 -> MATLAB Function1/1(WP)
  WPID/1 -> MATLAB Function1/2(WPID)  "WPID"
  Constant1/1 -> MATLAB Function1/3(P0)

== system PathFollowing_4_29/Waypoint Switch/Triggered Subsystem ==
  In1 : Inport
  Trigger : TriggerPort  TriggerType=falling  VariantControl=Variant
  WPID : Outport  InitialOutput=1
  wires:
  In1/1 -> WPID/1

== matlab function PathFollowing_4_29/plot ==
  data: x input size=1; y input size=1; psi input size=1
function drawship(x,y,psi)

coder.extrinsic("shipplot");
shipplot(x,y,psi)

== matlab function PathFollowing_4_29/Subsystem3/rudder1 ==
  data: alf input; u input; taorud_u output; v input; taorud_v output; taorud_r output
function [taorud_u,taorud_v,taorud_r]= rudder(alf,u,v)
C_b=0.53;w_R0=0.25;rou=1024;A_R=0.0025;lum_R=2.5;B=0.29;L=1.255;x_g=0.046;
V_rubber=sqrt(u^2+v^2);
f_a=6.13*lum_R/(2.25+lum_R);
t_R=0.2618+0.0539*C_b-0.1755*C_b^2;
a_H=0.6874-1.3374*C_b+1.8891*C_b^2;

if u==0
F_N=0;
else

% F_N=-rou*V_rubber^2*A_R*f_a*sin(a_r);
% V_rubber=U*(1-w_R)*sqrt(1+K_R*G_R);

gama=-2.22*(C_b*B/L)^2+0.02*C_b*B/L+0.68;
F_N=-rou*V_rubber^2*A_R*f_a*sin(alf-gama*(alf))/2;

end
taorud_u=(1-t_R)*F_N*sin(alf);
taorud_v=(1+a_H)*F_N*cos(alf)*sign(alf);
taorud_r=L/2*abs(F_N)*cos(alf)*sign(alf);
end

== matlab function PathFollowing_4_29/Waypoint Switch/If Action Subsystem1/MATLAB Function1 ==
  data: dx output; WP input; dy output; WPID input; Gamma_p output; P0 input
function [dx,dy,Gamma_p] = fcn(WP,WPID,P0)
dx = WP(WPID,1);
dy = WP(WPID,2);
if WPID == 1
    Gamma_p = atan2(dy-P0(2),dx-P0(1));
else
    Gamma_p = atan2(dy-WP(WPID-1,2),dx-WP(WPID-1,1));
end
if Gamma_p<0
    Gamma_p = Gamma_p + 2*pi;
end

== matlab function PathFollowing_4_29/Track Error Cal ==
  data: ye output; x input; xe output; y input; x_d input; y_d input; Gamma_p input
function [ye,xe] = fcn(x,y,x_d,y_d,Gamma_p)
xe = (x_d-x)*cos(Gamma_p)+(y_d-y)*sin(Gamma_p);
ye = -(x_d-x)*sin(Gamma_p)+(y_d-y)*cos(Gamma_p);

== matlab function PathFollowing_4_29/Subsystem3/back_propell ==
  data: v_b input size=1; n input size=1; T output; Q output; lm0 output
function [T,Q,lm0] = TMAU5(v_b,n)
%MAU5 计算MAU5叶桨的推力系数和扭矩系数
%   输入盘面比area_ratio
%   输入螺距比pitch_ratio
%   输入进速系数JA
area_ratio=0.65;
P=0.280;%螺距
D=0.2;%直径
omg=0.12;
rou=1024;
pitch_ratio=P/D;
% v_b=0.2;
% n=40;
% P/D=0.14
JA=(1-omg)*v_b/(n*D);
[~,column]=size(JA);


JA1=repmat(JA,16,1); %将JA构造成计算KT的列向量
JA2=repmat(JA,23,1); %将JA构造成计算KQ*10的列向量
[~,columnpitch_ratio]=size(pitch_ratio);
KT2=zeros(16,1);KQ102=zeros(23,1);

for i=1:column
KTData=[0.0536701800000000,0,0,0;-0.302356600000000,0,0,1;0.433362500000000,0,1,0;-0.106547100000000,1,0,2;-0.658290400000000,3,2,0;0.118910100000000,1,1,3;-0.000440856000000000,0,6,0;-0.0331785700000000,1,1,4;1.15112400000000,2,2,0;0.196077300000000,3,0,0;-0.0974706200000000,1,3,0;0.203638400000000,0,1,1;-0.256615300000000,1,1,1;-0.137024200000000,0,0,2;-0.287429400000000,2,0,0;-0.285160900000000,1,2,0];
KQ10Data=[-0.0925139000000000,0,0,0;-0.122900000000000,0,2,0;0.305069700000000,0,1,1;-0.293530300000000,0,0,2;-0.399147400000000,1,2,0;-1.02205000000000,1,1,1;0.0102283300000000,0,7,0;0.00352110000000000,3,1,0;0.00255205900000000,0,5,0;0.214353200000000,3,0,1;0.000713111000000000,0,4,4;0.207848800000000,1,1,2;0.639705800000000,0,1,0;0.000940485000000000,0,7,1;-0.0293004400000000,1,0,1;-0.0780762300000000,0,0,4;-0.302552300000000,3,2,2;0.185510500000000,1,1,3;-0.672421000000000,2,2,1;-0.208714200000000,3,4,0;0.940065400000000,1,3,0;0.931634600000000,3,2,1;-0.0434839700000000,0,6,0];
area_ratio1=(linspace(area_ratio,area_ratio,16))';        %将输入的盘面比转为列向量,用于计算KT
pitch_ratio1=(linspace(pitch_ratio(:,1),pitch_ratio(:,1),16))';     %将输入的螺距比转为列向量,用于计算KT
area_ratio2=(linspace(area_ratio,area_ratio,23))';        %将输入的盘面比转为列向量,用于计算KQ10
pitch_ratio2=(linspace(pitch_ratio(:,1),pitch_ratio(:,1),23))';     %将输入的螺距比转为列向量,用于计算KQ10                           
KT1=[area_ratio1.^KTData(:,2),pitch_ratio1.^KTData(:,3),JA1(:,i).^KTData(:,4)];  %构造KT盘面比、螺距比、进速系数次方矩阵
KQ101=[area_ratio2.^KQ10Data(:,2),pitch_ratio2.^KQ10Data(:,3),JA2(:,i).^KQ10Data(:,4)];  %构造KT盘面比、螺距比、进速系数次方矩阵
KT2(:,i)=[KTData(:,1).*KT1(:,1).*KT1(:,2).*KT1(:,3)];
KQ102(:,i)=[KQ10Data(:,1).*KQ101(:,1).*KQ101(:,2).*KQ101(:,3)];
end

KT3=sum(KT2);
KQ103=sum(KQ102);
KT=KT3;
KQ10=KQ103;
% KT=0.256265288489963;
% KQ10=0.300110834595595;

%推力
T=rou*n^2*D^4*KT;
Q=rou*n^2*D^5*KQ10/10;

lm0=10*KT*JA/KQ10/2/pi;


end

== matlab function PathFollowing_4_29/Kinematics /MATLAB Function ==
  data: flowDir input; u_c output; flowVel input; yaw input; u_v output
function [u_c,u_v] = fcn(flowDir,flowVel,yaw)
dAngle = flowDir-yaw;
if dAngle > 2*pi
    dAngle = dAngle-2*pi;
elseif dAngle<0
    dAngle = dAngle+2*pi;
end
u_c = flowVel*cos(dAngle);
u_v = flowVel*sin(dAngle);

== matlab function PathFollowing_4_29/Subsystem3/T2tor ==
  data: T input size=1; tor_r output
function tor_r = T_tao(T)
L=1.225;
tor_r=L*T/2;

end

== matlab function PathFollowing_4_29/Subsystem3/bow_thrust ==
  data: v_b input size=1; n input size=1; T output; Q output; lm0 output
function [T,Q,lm0] = TMAU5(v_b,n)
%MAU5 计算MAU5叶桨的推力系数和扭矩系数
%   输入盘面比area_ratio
%   输入螺距比pitch_ratio
%   输入进速系数JA
area_ratio=0.65;
pitch_ratio=0.7;
P=0.0280;%螺距
D=0.02;%直径
omg=0.12;
rou=1024;
% v_b=0.2;
% n=40;
% P/D=0.7
JA=(1-omg)*v_b/(n*D);
[~,column]=size(JA);
lm0=0;
if n==0
KT=0;
KQ10=0;
else
JA1=repmat(JA,16,1); %将JA构造成计算KT的列向量
JA2=repmat(JA,23,1); %将JA构造成计算KQ*10的列向量
[~,columnpitch_ratio]=size(pitch_ratio);
KT2=zeros(16,1);KQ102=zeros(23,1);

for i=1:column
KTData=[0.0536701800000000,0,0,0;-0.302356600000000,0,0,1;0.433362500000000,0,1,0;-0.106547100000000,1,0,2;-0.658290400000000,3,2,0;0.118910100000000,1,1,3;-0.000440856000000000,0,6,0;-0.0331785700000000,1,1,4;1.15112400000000,2,2,0;0.196077300000000,3,0,0;-0.0974706200000000,1,3,0;0.203638400000000,0,1,1;-0.256615300000000,1,1,1;-0.137024200000000,0,0,2;-0.287429400000000,2,0,0;-0.285160900000000,1,2,0];
KQ10Data=[-0.0925139000000000,0,0,0;-0.122900000000000,0,2,0;0.305069700000000,0,1,1;-0.293530300000000,0,0,2;-0.399147400000000,1,2,0;-1.02205000000000,1,1,1;0.0102283300000000,0,7,0;0.00352110000000000,3,1,0;0.00255205900000000,0,5,0;0.214353200000000,3,0,1;0.000713111000000000,0,4,4;0.207848800000000,1,1,2;0.639705800000000,0,1,0;0.000940485000000000,0,7,1;-0.0293004400000000,1,0,1;-0.0780762300000000,0,0,4;-0.302552300000000,3,2,2;0.185510500000000,1,1,3;-0.672421000000000,2,2,1;-0.208714200000000,3,4,0;0.940065400000000,1,3,0;0.931634600000000,3,2,1;-0.0434839700000000,0,6,0];
area_ratio1=(linspace(area_ratio,area_ratio,16))';        %将输入的盘面比转为列向量,用于计算KT
pitch_ratio1=(linspace(pitch_ratio(:,1),pitch_ratio(:,1),16))';     %将输入的螺距比转为列向量,用于计算KT
area_ratio2=(linspace(area_ratio,area_ratio,23))';        %将输入的盘面比转为列向量,用于计算KQ10
pitch_ratio2=(linspace(pitch_ratio(:,1),pitch_ratio(:,1),23))';     %将输入的螺距比转为列向量,用于计算KQ10                           
KT1=[area_ratio1.^KTData(:,2),pitch_ratio1.^KTData(:,3),JA1(:,i).^KTData(:,4)];  %构造KT盘面比、螺距比、进速系数次方矩阵
KQ101=[area_ratio2.^KQ10Data(:,2),pitch_ratio2.^KQ10Data(:,3),JA2(:,i).^KQ10Data(:,4)];  %构造KT盘面比、螺距比、进速系数次方矩阵
KT2(:,i)=[KTData(:,1).*KT1(:,1).*KT1(:,2).*KT1(:,3)];
KQ102(:,i)=[KQ10Data(:,1).*KQ101(:,1).*KQ101(:,2).*KQ101(:,3)];
end

KT3=sum(KT2);
KQ103=sum(KQ102);
KT=KT3;
KQ10=KQ103;
% KT=0.256265288489963;
% KQ10=0.300110834595595;
lm0=10*KT*JA/KQ10/2/pi;
end
%推力
T=rou*n^2*D^4*KT*sign(n);
Q=rou*n^2*D^5*KQ10/10*sign(n);




end

== matlab function PathFollowing_4_29/Subsystem/wave/wave ==
  data: K_w1 output; K_w2 output; K_w3 output; u_wind input; v_wind input; r_wind input
function [K_w1,K_w2,K_w3] = wave(u_wind,v_wind,r_wind)
%pra
w_0=1.1;
lamda=0.1017;
w_e1=0.8;w_e2=0.8;w_e3=0.8;
A=8.1*10e-3*9.81^2;%A cons
B1=0.74*(0.81/u_wind)^4;
delta1=sqrt((A/w_0^5)*exp(-B1/w_0^4));
K_w1=2*lamda*w_0*delta1;%gain constant1
B2=0.74*(0.81/v_wind)^4;
delta2=sqrt((A/w_0^5)*exp(-B2/w_0^4));
K_w2=2*lamda*w_0*delta2;%gain constant2
B3=0.74*(0.81/r_wind)^4;
delta3=sqrt((A/w_0^5)*exp(-B3/w_0^4));
K_w3=2*lamda*w_0*delta3;%gain constant3

end
